simulink model "Solar_MPPT_Resistaince_load_p_o_cuk"  (Simulink 8.1)
settings: Solver=ode45  StartTime=0.0  StopTime=.01  RelTol=1e-3
libraries: powerlib x15, simulink x1
settings Model: Creator=Goal-Kartik  LastModifiedBy=Kartik
settings DebuggingCC: FcnCallInpInsideContextMsg=EnableAllAsWarning
settings GRTTargetCC: CombineOutputUpdateFcns=on  GRTInterface=off

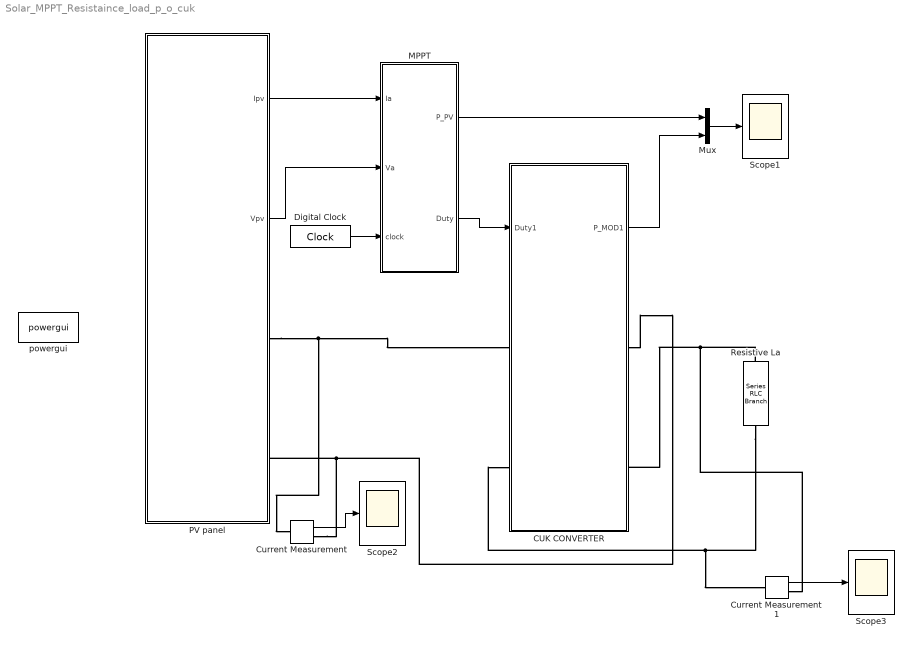
== system Solar_MPPT_Resistaince_load_p_o_cuk ==
  CUK CONVERTER : Subsystem
  Current Measurement : powerlib/Measurements/Current Measurement  PhasorSimulation=off  OutputType=Complex  PSBequivalent=0
  Current Measurement1 : powerlib/Measurements/Current Measurement  PhasorSimulation=off  OutputType=Complex  PSBequivalent=0
  Digital Clock : DigitalClock  SampleTime=0.001
  MPPT : Subsystem
  Mux : Mux  Inputs=2
  PV panel : Subsystem
  Resistive La : powerlib/Elements/Series RLC Branch  LConnTagsString=__new0  RConnTagsString=__new0  BranchType=R  Resistance=30  Inductance=1e-3  SetiL0=off  InitialCurrent=0  Capacitance=1e-6  Setx0=off  InitialVoltage=0  Measurements=None
  Scope1 : Scope
      settings: TimeRange=0.01  YMin=-50  YMax=350  SaveName=ScopeData2
  Scope2 : Scope
      settings: TimeRange=0.01  YMin=-50  YMax=350
  Scope3 : Scope
      settings: TimeRange=0.01  YMin=-50  YMax=350  SaveName=ScopeData3
  powergui : powerlib/powergui  SimulationMode=Discrete  SolverType=Tustin  SampleTime=1e-6  frequency=60  SPID=off  DisableSnubberDevices=off  DisableRonSwitches=off  DisableVfSwitches=off  SwTol=0  Interpol=off  DisplayEquations=off  frequencyindice=0  Pbase=100e6  ErrMax=1e-4  Iterations=50  UnitsV=kV  UnitsW=MW  FunctionMessages=off  echomessages=off  HookPort=off  EnableUseOfTLC=off  x0status=blocks  RestoreLinks=warning  ResistiveCurrentMeasurement=off  Frange=[0:2:500]  Ylog=off  Xlog=on  ShowGrid=off  save=off  variable=ZData  structure=ScopeData  ZoomFFT=off  StartTime=0.04  cycles=2  DisplayStyle=1  fundamental=1000  FreqAxis=off  MaxFrequency=50000  frequencyindicesteady=1  RmsSteady=1  display=off  Ts=0  methode=off
  wires:
  PV panel/1(Ipv) -> MPPT/1(Ia)
  PV panel/2(Vpv) -> MPPT/2(Va)
  Digital Clock/1 -> MPPT/3(clock)
  MPPT/1(P_PV) -> Mux/1
  Mux/1 -> Scope1/1
  MPPT/2(Duty) -> CUK CONVERTER/1(Duty1)
  CUK CONVERTER/1(P_MOD1) -> Mux/2
  Current Measurement/1 -> Scope2/1
  Current Measurement1/1 -> Scope3/1
  connections:
  Current Measurement/LConn1 -- PV panel/RConn1 -- CUK CONVERTER/LConn1
  CUK CONVERTER/RConn1 -- PV panel/RConn2 -- Current Measurement/RConn1
  Resistive La/LConn1 -- CUK CONVERTER/RConn2 -- Current Measurement1/RConn1
  Resistive La/RConn1 -- CUK CONVERTER/LConn2 -- Current Measurement1/LConn1

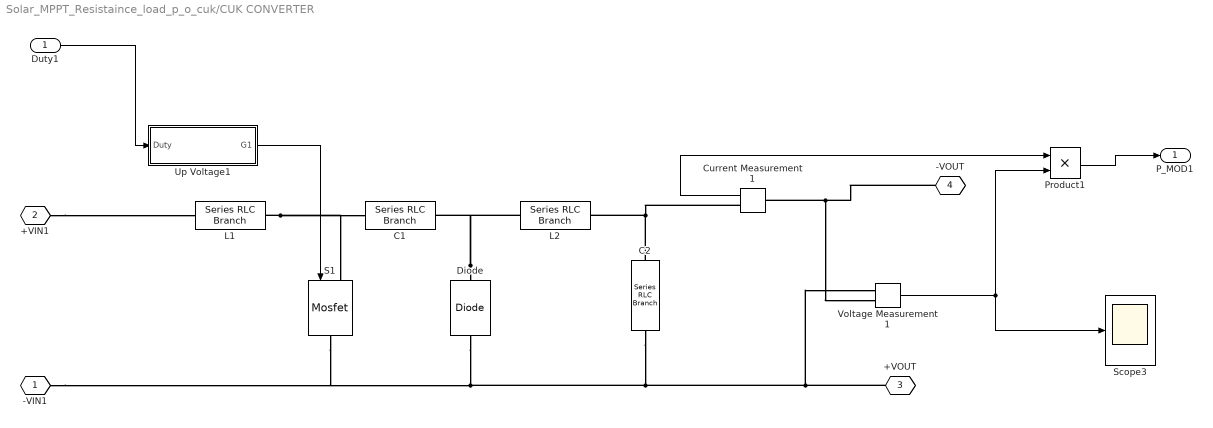
== system Solar_MPPT_Resistaince_load_p_o_cuk/CUK CONVERTER ==
  Duty1 : Inport
  C1 : powerlib/Elements/Series RLC Branch  LConnTagsString=__new0  RConnTagsString=__new0  BranchType=C  Resistance=1  Inductance=1e-3  SetiL0=off  InitialCurrent=0  Capacitance=200e-6  Setx0=off  InitialVoltage=0  Measurements=Branch voltage and current
  C2 : powerlib/Elements/Series RLC Branch  LConnTagsString=__new0  RConnTagsString=__new0  BranchType=C  Resistance=1  Inductance=1e-3  SetiL0=off  InitialCurrent=0  Capacitance=220e-6  Setx0=off  InitialVoltage=0  Measurements=Branch current
  Current Measurement1 : powerlib/Measurements/Current Measurement  PhasorSimulation=off  OutputType=Complex  PSBequivalent=0
  Diode : powerlib/Power Electronics/Diode  Ron=0.001  Lon=0  Vf=0.8  IC=0  UseSnubber=off  Rs=500  Cs=250e-9  Measurements=off
  L1 : powerlib/Elements/Series RLC Branch  LConnTagsString=__new0  RConnTagsString=__new0  BranchType=L  Resistance=1  Inductance=180e-6  SetiL0=off  InitialCurrent=0  Capacitance=1e-6  Setx0=off  InitialVoltage=0  Measurements=Branch voltage and current
  L2 : powerlib/Elements/Series RLC Branch  LConnTagsString=__new0  RConnTagsString=__new0  BranchType=L  Resistance=1  Inductance=150e-6  SetiL0=off  InitialCurrent=0  Capacitance=1e-6  Setx0=off  InitialVoltage=0  Measurements=Branch voltage and current
  Product1 : Product  RndMeth=Zero
  S1 : powerlib/Power Electronics/Mosfet  Ron=0.1  Lon=0  Rd=0.01  Vfd=0  IC=0  Rs=1e5  Cs=inf  Measurements=off
  Scope3 : Scope
      settings: TimeRange=1  YMin=63.35  YMax=64.2  SaveName=ScopeData5
  Up Voltage1 : Subsystem  mask{fc=10000, Gama=0.5}
      mask prompts: fc "Frequency (Hz)"; Gama "Duty Cycle  (0-1)"
      mask Display: disp('CONTROL SIGNAL')
  Voltage Measurement1 : powerlib/Measurements/Voltage Measurement  PhasorSimulation=off  OutputType=Complex  PSBequivalent=0
  -VIN1 : PMIOPort  Tag=PMCPort  Port=1  Side=Right
  +VIN1 : PMIOPort  Tag=PMCPort  Port=2  Side=Left
  +VOUT : PMIOPort  Tag=PMCPort  Port=3  Side=Right
  -VOUT : PMIOPort  Tag=PMCPort  Port=4  Side=Left
  P_MOD1 : Outport
  wires:
  ? -> ?
  Duty1/1 -> Up Voltage1/1(Duty)
  Up Voltage1/1(G1) -> S1/1
  Current Measurement1/1 -> Product1/1
  Voltage Measurement1/1 -> Scope3/1, Product1/2
  Product1/1 -> P_MOD1/1
  connections:
  L1/RConn1 -- S1/LConn1 -- C1/LConn1
  +VOUT/RConn1 -- C2/RConn1 -- S1/RConn1 -- -VIN1/RConn1 -- Diode/RConn1 -- Voltage Measurement1/LConn1
  Diode/LConn1 -- L2/LConn1 -- C1/RConn1
  C2/LConn1 -- L2/RConn1 -- Current Measurement1/RConn1
  +VIN1/RConn1 -- L1/LConn1
  -VOUT/RConn1 -- Current Measurement1/LConn1 -- Voltage Measurement1/LConn2

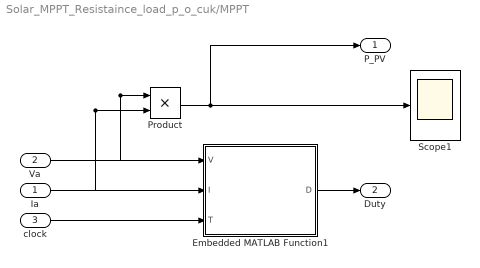
== system Solar_MPPT_Resistaince_load_p_o_cuk/MPPT ==
  Ia : Inport
  Va : Inport  Port=2
  clock : Inport  Port=3
  Embedded MATLAB Function1 : MATLAB Function  TreatAsAtomicUnit=on
  Product : Product  RndMeth=Zero
  Scope1 : Scope
      settings: TimeRange=0.09  YMin=158.4  YMax=159.4  SaveName=ScopeData4
  P_PV : Outport
  Duty : Outport  Port=2
  wires:
  Ia/1 -> Product/2, Embedded MATLAB Function1/2(I)
  Va/1 -> Embedded MATLAB Function1/1(V), Product/1
  clock/1 -> Embedded MATLAB Function1/3(T)
  Product/1 -> Scope1/1, P_PV/1
  Embedded MATLAB Function1/1(D) -> Duty/1

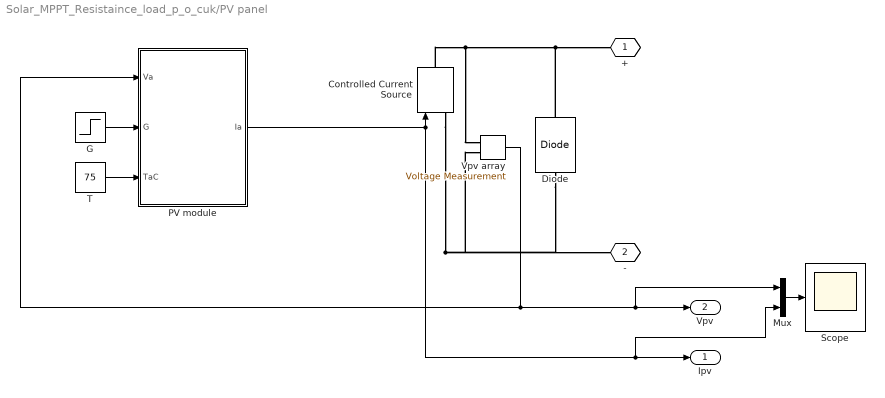
== system Solar_MPPT_Resistaince_load_p_o_cuk/PV panel ==
  Controlled Current Source : powerlib/Electrical Sources/Controlled Current Source  Initialize=on  Source_Type=AC  Amplitude=0  Phase=0  Frequency=0  Measurements=None
  Diode : powerlib/Power Electronics/Diode  Ron=0.001  Lon=0  Vf=0  IC=0  UseSnubber=off  Rs=500  Cs=250e-9  Measurements=off
  G : Step  Time=0  SampleTime=0
  Mux : Mux  Inputs=2
  PV module : MATLAB Function  TreatAsAtomicUnit=on
  Scope : Scope
      settings: TimeRange=0.09999999999999999  YMin=9  YMax=27
  T : Constant  Value=75
  Vpv array : powerlib/Measurements/Voltage Measurement  PhasorSimulation=off  OutputType=Complex  PSBequivalent=0
  + : PMIOPort  Tag=PMCPort  Port=1  Side=Right
  - : PMIOPort  Tag=PMCPort  Port=2  Side=Right
  Ipv : Outport
  Vpv : Outport  Port=2
  wires:
  G/1 -> PV module/2(G)
  T/1 -> PV module/3(TaC)
  PV module/1(Ia) -> Controlled Current Source/1, Ipv/1, Mux/2
  Vpv array/1 -> PV module/1(Va), Vpv/1, Mux/1
  Mux/1 -> Scope/1
  connections:
  Controlled Current Source/LConn1 -- Diode/LConn1 -- -/RConn1 -- Vpv array/LConn2
  Controlled Current Source/RConn1 -- Diode/RConn1 -- +/RConn1 -- Vpv array/LConn1

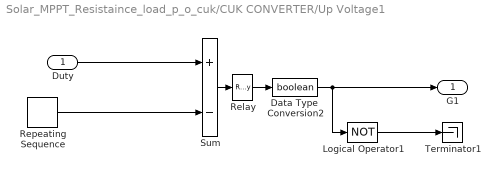
== system Solar_MPPT_Resistaince_load_p_o_cuk/CUK CONVERTER/Up Voltage1 ==
  Duty : Inport
  Data Type  Conversion2 : DataTypeConversion  OutDataTypeStr=boolean  SaturateOnIntegerOverflow=on  RndMeth=Zero
  Logical Operator1 : Logic  Operator=NOT
  Relay : Relay
  Repeating Sequence : simulink/Sources/Repeating Sequence  rep_seq_t=[0 1/10e3]  rep_seq_y=[0 1]
  Sum : Sum  Inputs=+-  SaturateOnIntegerOverflow=on  InputSameDT=on  OutDataTypeStr=Inherit: Same as first input
  Terminator1 : Terminator
  G1 : Outport
  wires:
  Logical Operator1/1 -> Terminator1/1
  Relay/1 -> Data Type  Conversion2/1
  Sum/1 -> Relay/1
  Repeating Sequence/1 -> Sum/2
  Duty/1 -> Sum/1
  Data Type  Conversion2/1 -> G1/1, Logical Operator1/1

== matlab function MPPT/Embedded MATLAB Function1 ==
  data: V input double; I input double; T input double; D output double
function D   = PO(V,I,T)
persistent P2  P1  dP d dd n;
if isempty(V)
    V=20;
end
if isempty(I)
    I=0;
end
if isempty(P2)
    P2=0;
end
if isempty(P1)
    P1=0;
end
if isempty(dP)
    dP=0;
end
if isempty(d)
    d=1;
end
if isempty(dd)
    dd=0;
end
if isempty(n)
    n=1;
end
%%%%%%%%%%%%%%%%%%%%%
    if  (T > n*0.02)   %chu ki lay mau 0.02s
    n = n + 1;
    P1=P2;
    P2=V*I;
    dP=P2-P1;
    if (dd==0)
        if dP>1
            dd=0.01;
            d=d+dd;
        else
            if dP<-1
                dd=-0.01;
                d=d+dd;
            else
                dd=0;
            end
        end
    else
        if ((dP<1)&&(dP>-1))
        dd=0;
        d=d+dd;
        else
            if ((dP/dd)>0)
                dd=0.01;
                d=d+dd;
            else
                dd=-0.01;
                d=d+dd;
            end
        end
    end    
    end
D=d/(d+1);
if D<0.1
    D=0.1;
    d=D/(1-D);
else
    if D>0.9
        D=0.9;
        d=D/(1-D);
    else
    end
end
end

== matlab function PV panel/PV module ==
  data: Va input double; Ia output double; G input double; TaC input double
function Ia=Iphoton(Va,G,TaC) 

% Out: Ia = Module operating current (A)
% In:  Va = Module operating voltage (V)
%      G = Do roi (1G = 1000 W/m^2)
%      TaC = (celsius)

%----------------------------------------------------------------------
k = 1.381e-23;      %  Boltzmann  
q = 1.602e-19;      %  electron charge 
n = 1.3;           %  (1<n<2)
Eg = 1.12;          %  1.12eV (Si), 1.42 (GaAs) 
Ns = 10;            %  cell 
Np=6;
TrK = 298;          %25  C
Voc_TrK = 37.51 /Ns; % Voc :  25 C 
Isc_TrK = 8.63/Np;     % Isc:   25  C                                             
a = 1.33e-3;        % He  (0.065A/C) 
TaK = 273 + TaC;     % temp
Vc = Va / Ns;       %  cell 

Isc = Isc_TrK * (1 + (a * (TaK - TrK))); 
%  G( G=1KW/m2)
Iph = G * Isc;  
% temp 25  C 
Vt_TrK = n * k * TrK / q;    
%  b = Eg * q/(n*k) 
b = Eg * q /(n * k); 

Ir_TrK = Isc_TrK / (exp(Voc_TrK / Vt_TrK) -1); 
Ir = Ir_TrK * (TaK / TrK)^(3/n) * exp(-b * (1 / TaK -1 / TrK)); 

dVdI_Voc = -2.0/Ns;    % Take dV/dI @ Voc from I-V curve of datasheet 
Xv = Ir_TrK / Vt_TrK * exp(Voc_TrK / Vt_TrK); 
Rs = - dVdI_Voc - 1/Xv;   
% The temp
Vt_Ta = n * k * TaK / q;                                                          
% Ia = Iph - Ir * (exp((Vc + Ia * Rs) / Vt_Ta) -1) 
% f(Ia) = Iph - Ia - Ir * ( exp((Vc + Ia * Rs) / Vt_Ta) -1) = 0 
% Solve for Ia by Newton's method: Ia2 = Ia1 - f(Ia1)/f'(Ia1) 
Ia=zeros(size(Vc)); % Initialize Ia with zeros   
for j=1:5; 
    Ia = Ia - (Iph - Ia - Ir .* ( exp((Vc + Ia .* Rs) ./ Vt_Ta) -1))... 
        ./ (-1 - Ir * (Rs ./ Vt_Ta) .* exp((Vc + Ia .* Rs) ./ Vt_Ta)); 
end
Ia=Ia*Np;
end
